simulink model "RoboBoatVU_2014_Final_Run"  (R2014a)
settings: Solver=FixedStepDiscrete  StartTime=0.0  StopTime=inf  FixedStep=.1  RelTol=1e-3
undefined symbols (not defined in the file): Com1, Com2, Com3, Com4, DiscIntNeverNeededParam, RGB24, standard
libraries: visiontextngfix x66, simulink x53, xpcseriallib x15, dspmtrx3 x14, slrtlib x3, speedgoatlib_IO102 x3, visionstatistics x2, dspstat3 x2, dspindex x2, xpcvideousblib x2, xpcvideoutillib x2, speedgoatlib x1
(part 7 of 7)

== matlab function RoboBoatVU_2014_Final_Run/Main FSM/Obstacle Navigation1/Enter Gate/Gate 2 (White & White)/MATLAB Function ==
  data: Prob input; RPM output; ColorID input; Dist input; Ang input; CurrentHeading input; GPSLat input; GPSLong input; Timer input; DesiredHeading output; gateGPS output
function [RPM,DesiredHeading,gateGPS] = navigation(Prob,ColorID,Dist,Ang,CurrentHeading,GPSLat,GPSLong,Timer)

% Function performs one buoy navigation through the start speed gates. If
% no buoys are found by the LIDAR/Vision assembly then an incremented
% turning algorithm is executed to turn by 10 degrees per increment up to 
% 90 degrees either way of the inital heading

% Written by Edward Zhu


persistent LockHeading TimeLastFound Counter Turn TurnInc gateLat gateLong

if isempty(LockHeading) && isempty(TimeLastFound) && isempty(Counter) && isempty(Turn) && isempty(TurnInc)
    LockHeading = CurrentHeading;
    TimeLastFound = 0;
    Counter = 0;
    TurnInc = 30;
    Turn = TurnInc;
    gateLat = 0;
    gateLong = 0;
end
Distance = Dist/100;
BoatWidth = 0.75;
Buffer = atan(2*BoatWidth/Distance);

RedOffset = Ang + Buffer;
WhiteOffset = Ang - Buffer;

R = 6378137;

CurLat = (floor(GPSLat/100)+mod(GPSLat,100)/60)*pi/180;
CurLong = (ceil(GPSLong/100)-mod(-GPSLong,100)/60)*pi/180;

gateHeading = (mod(CurrentHeading - Ang, 360))*pi/180;

if ColorID == 1 && Prob > 0.9
    DesiredHeading = mod(CurrentHeading - RedOffset, 360);
    RPM = 2000;
    GateFound = 1;
    TimeLastFound = Timer;
    gateLat =  asin(sin(CurLat)*cos(Distance/R) + cos(CurLat)*sin(Distance/R)*cos(gateHeading))*180/pi;
    gateLong = (CurLong + atan2(sin(gateHeading)*sin(Distance/R)*cos(CurLat),cos(Distance/R)-sin(CurLat)*sin(gateLat)))*180/pi;
elseif ColorID == 2 && Prob > 0.9
    DesiredHeading = mod(CurrentHeading - WhiteOffset, 360);
    RPM = 2000;
    GateFound = 1;
    TimeLastFound = Timer;
    gateLat =  asin(sin(CurLat)*cos(Distance/R) + cos(CurLat)*sin(Distance/R)*cos(gateHeading))*180/pi;
    gateLong = (CurLong + atan2(sin(gateHeading)*sin(Distance/R)*cos(CurLat),cos(Distance/R)-sin(CurLat)*sin(gateLat)))*180/pi;
else
    DesiredHeading = CurrentHeading;
    RPM = 0;
    GateFound = 0;
end

gateGPS = [gateLat gateLong];
TimeNoBuoys = Timer - TimeLastFound;

if GateFound == 0 && TimeNoBuoys > 15
    RPM = 0;
    DesiredHeading = mod(LockHeading - Turn, 360);
    HeadingDiff = DesiredHeading - CurrentHeading;
    gateGPS = [gateLat gateLong];
    
    if HeadingDiff > 180
        HeadingDiff = HeadingDiff - 360;
    elseif HeadingDiff < -180
        HeadingDiff = HeadingDiff + 360;
    end
    
    if HeadingDiff < 3
        Counter = Counter + 1;
    else
        Counter = 0;
    end
    
    if Counter >= 15
        Turn = Turn + TurnInc;
        Counter = 0;
        if abs(Turn) > 90
            TurnInc = -TurnInc;
        end
    end
end

== matlab function RoboBoatVU_2014_Final_Run/Main FSM/Obstacle Navigation1/GPS: Center/GPS Enabler ==
  data: Finished input; GPSMode output; OrientEnable output; ApproachEnable output
function [GPSMode, OrientEnable, ApproachEnable] =...
    GPSEnable(Finished)

%Written by Anderson Lebbad on July 22, 2013
%Last Edited: July 27, 2013
%   Removed Termination Block

%This function enables GPS tasks. First the boat orients towards the
%target, then it approaches it.


%Parse Finished signal
OrientFinished = Finished(1);


%Initialize Enablers
OrientEnable = 0;
ApproachEnable = 0;


%Switches the enable signal based on which task is flagged as done.
if OrientFinished == 0
    OrientEnable = 1;
    GPSMode = 1;
else
    ApproachEnable = 1;
    GPSMode = 2;
end

== matlab function RoboBoatVU_2014_Final_Run/Main FSM/Obstacle Navigation1/Obstacle Navigation/Dodge/Nav Logic ==
  data: CurrentHeading input; Dist input; Ang input; ObstDist output; RPM output; DesiredHeading output; Timer input; Timeout input; DodgeIncomplete output
 function [ObstDist, RPM, DesiredHeading, DodgeIncomplete] = NavLogic(CurrentHeading,...
    Dist, Ang, Timer, Timeout)

%Written by Anderson Lebbad on August 20, 2013
%Last Edited by:

%Determines the signals for driving through the buoy channel based on the
%bounding box and centroid signals from both the red and green detection
%blocks.

persistent TimeLastFound heldHeading

ObstDist = Dist / 100;

if isempty(TimeLastFound) && isempty(heldHeading)
    TimeLastFound = 0;
    heldHeading = CurrentHeading;
end

if ObstDist > 0 && ObstDist <= 2
    %Buffer for single buoy offset is the angle to twice the boat's width off of the
    %center of the buoy
    BoatWidth = .75;
    Buffer = atan(2 * BoatWidth / ObstDist) * 180 / pi;
    
    if Ang < 0
        ObstOffset = Ang + Buffer;
    else
        ObstOffset = Ang - Buffer;
    end
    
    DesiredHeading = mod(CurrentHeading + ObstOffset, 360);
    RPM = 2800;
    
    TimeLastFound = Timer;
    heldHeading = CurrentHeading;
    
    DodgeIncomplete = 1;
    
else
    DesiredHeading = heldHeading;
    RPM = 2800;
    
    if Timer-TimeLastFound < Timeout
        DodgeIncomplete = 1;
    else
        DodgeIncomplete = 0;
    end

end

== matlab function RoboBoatVU_2014_Final_Run/Main FSM/Obstacle Navigation1/Obstacle Navigation/GPS: Bee Line/Orient/Within Range ==
  data: DesiredHeading input; Finished output; Compass input
function Finished = OrientLocked(DesiredHeading, Compass)

%Written by Anderson Lebbad on July 22, 2013
%Last Edited:

%This function checks to see if the target heading has been reached and 
%sends a finished signal when it has.

HeadingDiff = DesiredHeading - Compass;

%Sets the range for the difference angle to be -180 to +180
if HeadingDiff > 180
    HeadingDiff = HeadingDiff - 360;
elseif HeadingDiff < -180
    HeadingDiff = HeadingDiff + 360;
end

%If the Heading is within 3 degrees, the angle is close enough to send a
%finished signal
if abs(HeadingDiff) < 3
    Finished = 1;
else
    Finished = 0;
end

== matlab function RoboBoatVU_2014_Final_Run/Main FSM/Shotgun Speedgate/MATLAB Function ==
  data: Heading input; LockedHeading output
function LockedHeading = HeadingLock(Heading)

persistent lock

if isempty(lock)
    lock = Heading;
end

LockedHeading = lock;

== matlab function RoboBoatVU_2014_Final_Run/Parameters/GPS Points/GPS Selector ==
  data: course input; ssGate output; rtnIn input; ssGateA input; transWptA input; obstNavStartA input; obstNavEndA input; acouLocA input; dockA input; ssGateB input; transWptB input; obstNavStartB input; obstNavEndB input; acouLocB input; dockB input; ssGateT input; transWptT input; obstNavStartT input; obstNavEndT input; acouLocT input; dockT input; transWpt output; obstNavStart output; obstNavEnd output; acouLoc output; dock output; rtnOut output
function [ssGate,transWpt,obstNavStart,obstNavEnd,acouLoc,dock,rtnOut] = ...
    GPSselector(course,rtnIn,...
    ssGateA,transWptA,obstNavStartA,obstNavEndA,acouLocA,dockA,...
    ssGateB,transWptB,obstNavStartB,obstNavEndB,acouLocB,dockB,...
    ssGateT,transWptT,obstNavStartT,obstNavEndT,acouLocT,dockT)

%Written by: Anderson Lebbad on July 18, 2013
%Last Edited: Edward Zhu on June
%   Data type mismatch addressed
%   Character conversion redundant

%Selects GPS Points to use based on input Course

%Check value of CourseStr and pass inputs accordingly

switch course
    case uint8('A')
        ssGate = ssGateA;
        transWpt = transWptA;
        obstNavStart = obstNavStartA;
        obstNavEnd = obstNavEndA;
        acouLoc = acouLocA;
        dock = dockA;
        rtnOut = rtnIn;
        
    case uint8('B')
        ssGate = ssGateB;
        transWpt = transWptB;
        obstNavStart = obstNavStartB;
        obstNavEnd = obstNavEndB;
        acouLoc = acouLocB;
        dock = dockB;
        rtnOut = rtnIn;
        
    otherwise
        ssGate = ssGateT;
        transWpt = transWptT;
        obstNavStart = obstNavStartT;
        obstNavEnd = obstNavEndT;
        acouLoc = acouLocT;
        dock = dockT;
        rtnOut = rtnIn;
end

== matlab function RoboBoatVU_2014_Final_Run/Main FSM/Acoustic Location1/GPS: Acoustic Center1/GPS Enabler ==
  data: Finished input; GPSMode output; OrientEn output; ApproachEn output
function [GPSMode, OrientEn, ApproachEn] = GPSEnable(Finished)

%Written by Anderson Lebbad on July 22, 2013
%Last Edited: July 27, 2013
%   Removed Termination Block

%This function enables GPS tasks. First the boat orients towards the
%target, then it approaches it.


%Parse Finished signal
OrientFinished = Finished(1);


%Initialize Enablers
OrientEn = 0;
ApproachEn = 0;


%Switches the enable signal based on which task is flagged as done.
if OrientFinished == 0
    OrientEn = 1;
    GPSMode = 1;
else
    ApproachEn = 1;
    GPSMode = 2;
end

== matlab function RoboBoatVU_2014_Final_Run/Main FSM/Acoustic Location1/GPS:Waypoint/Approach/Desired Heading and Distance ==
  data: Distance output; DesiredGPS input; DesiredHeading output; GPSLat input; GPSLong input
function [Distance, DesiredHeading] = Approach(DesiredGPS, GPSLat, GPSLong)

%Written by Anderson Lebbad on July 22, 2013
%Last Edited: Edward Zhu July 5, 2014

%Edit:
% Switched from great-circle distance formula to equirectangular approx and
%used mod for desired heading
% Changed calculation to use positve lat and negative long

%Orients the boat towards a target GPS point before approaching it.
%This is done to keep the approach angle minimal, so the approach
%algorithm does not circle the target and never reach it.

%Parse input GPS and convert angles to radians
CurLat = (floor(GPSLat/100)+mod(GPSLat,100)/60)*pi/180;
CurLong = (ceil(GPSLong/100)-mod(-GPSLong,100)/60)*pi/180;
DesLat = (floor(DesiredGPS(1)/100)+mod(DesiredGPS(1),100)/60)*pi/180;
DesLong = (ceil(DesiredGPS(2)/100)-mod(-DesiredGPS(2),100)/60)*pi/180;

%Difference between lats and longs
DiffLat = DesLat - CurLat;
MidLat = cos((CurLat + DesLat)/2);
DiffLong = DesLong - CurLong;

%Radius of the earth in meters
R = 6378137;

%Calculate distance using the great-circle distance formula
%Formula documented here:
%   http://www.movable-type.co.uk/scripts/latlong.html
% a = sin(DiffLat/2)^2+sin(DiffLong/2)^2*cos(CurLat)*cos(DesLat);
% c = 2*atan2(sqrt(a), sqrt(1-a));
% Distance = R*c;

%Calculating distance using equirectangular approximation since distances
%concerned are very small
a = DiffLong*MidLat;
b = DiffLat;
Distance = R*sqrt(a^2+b^2);

%Calculate initial bearing - formula documented here: 
%   http://www.movable-type.co.uk/scripts/latlong.html
y = sin(DiffLong)*cos(DesLat);
x = cos(CurLat)*sin(DesLat)-sin(CurLat)*cos(DesLat)*cos(DiffLong);
DesiredHeading = mod(atan2(y, x)*180/pi + 360, 360);

== matlab function RoboBoatVU_2014_Final_Run/Main FSM/Start Speed Gate/Buoy Decisions/Nav Logic ==
  data: Compass input; RedBBox input; GreenBBox input; RedCentroid input; GreenCentroid input; Course input; RedDist output; GreenDist output; RPM output; DesiredHeading output; Timer input; RedGain input; GreenGain input
function [RedDist, GreenDist, RPM, DesiredHeading] = NavLogic(Compass,...
    RedBBox, GreenBBox, RedCentroid, GreenCentroid, Course, Timer,RedGain,GreenGain)

%Written by Anderson Lebbad on August 20, 2013
%Last Edited by:

%Determines the signals for driving through the buoy channel based on the
%bounding box and centroid signals from both the red and green detection
%blocks.


%Initialize Outputs
RPM = 2800;
DesiredHeading = Compass;



%% First, calculate the distance each detected polyform A-0 buoy is.

%The buoy has a fixed diameter (m), the camera has a known field of view
%(which will be converted to radians for calculations) and the size of the
%frame (in pixels) is fixed
diameter = 0.3556;
FoV = 62*pi/180;
wFrame = 640;


%The bounding box passes the width of the found buoy in pixels
wRedBox = RedBBox(3);
wGreenBox = GreenBBox(3);


%The ratio of the widths in pixels corresponds to the ratio of the withs in
%meters, and the width of the frame in meters is equal to the angle of the
%field of view (in radians) multiplied by the distance it is away from the
%buoy
RedDist = (wFrame * diameter) / (wRedBox * FoV);
GreenDist = (wFrame * diameter) / (wGreenBox * FoV);



%% Second, determine angles to buoys and offset angles for steering

%Reference angle measured from bottom center of the frame (image
%coordinates are referenced to top left corner of image, with higher x
%values being more towards the right of the image, and higher y values
%being more towards the bottom of the image)
RedX = RedCentroid(1) - 320;
RedY = 480 - RedCentroid(2);
GreenX = GreenCentroid(1) - 320;
GreenY = 480 - GreenCentroid(2);


%Return angles in degrees
RedAngle = atan(RedX / RedY) * 180 / pi;
GreenAngle = atan(GreenX / GreenY) * 180 / pi;


%Buffer for single buoy offset is the angle to twice the boat's width off of the
%center of the buoy
BoatWidth = .75;
RedBuffer = atan(RedGain * BoatWidth / RedDist) * 180 / pi;
GreenBuffer = atan(GreenGain * BoatWidth / GreenDist) * 180 / pi;


%Red offset is to the right and green is to the left to stay within gates
RedOffset = RedAngle + RedBuffer;
GreenOffset = GreenAngle - GreenBuffer;



%% Third, determine whether both buoys are located and whether or not
%navigation can treat them as a pair.

%Check to see if a valid value was passed for the centroid for both the red
%and green blobs
if RedCentroid(1) == -1
    RedLocate = 0;
else
    RedLocate = 1;
end
if GreenCentroid(1) == -1
    GreenLocate = 0;
else
    GreenLocate = 1;
end


%if both are located and red is to the left of green, steer between the
%two. Otherwise, do appropriate one buoy navigation, or mark no buoys as
%found
if RedLocate == 1 && GreenLocate == 1
    if RedAngle < GreenAngle
        DesiredHeading = mod(Compass + (RedAngle + GreenAngle) / 2, 360);
        RPM = 4000;
    elseif Course == 'A'
        DesiredHeading = mod(Compass + RedOffset, 360);
    else
        DesiredHeading = mod(Compass + GreenOffset, 360);
    end
    buoysFound = 2;
elseif RedLocate == 1
    DesiredHeading = mod(Compass + RedOffset, 360);
    buoysFound = 1;
elseif GreenLocate == 1
    DesiredHeading = mod(Compass + GreenOffset, 360);
    buoysFound = 1;
else
    buoysFound = 0;
end


%% Fourth, search algorithm if no buoys are found. The search algorithm is
%designed to first hold the last heading for two seconds (in case lighting
%and focus caused the buoys to not be detected for a few frames), then to
%turn away from the last buoy position in the opposite direction of the
%other course by the angle of the field of view, and then towards the
%direction of the other course by the angle of the field of view. If a buoy
%is not found by the time this is done, the boat orients itself back in the
%direction that a buoy was last found, and slowly backs up.

%Set a persistent variables to track the last time a buoy was detected and
%heading it was at when it saw it.
persistent TimeLastFound
if isempty(TimeLastFound)
    TimeLastFound = Timer;
end
persistent HeadingLastFound
if isempty(HeadingLastFound)
    HeadingLastFound = Compass;
end


%Set a variable for tracking the time since the last buoy was found
% TimeNoBuoys = Timer - TimeLastFound;


%Set a variable for which way to initially turn during the search algorithm
%based on the course number
% if Course == 'B'
%     Turn = -FoV * 180 / pi;
% else
%     Turn = FoV * 180 / pi;
% end

%Check to see if no buoys are found, and how long it has been to determine
%what part of the search algorithm to run
if buoysFound == 0
    DesiredHeading = HeadingLastFound;
    RPM = 4000;
    %     elseif TimeNoBuoys < 20
    %         DesiredHeading = mod(HeadingLastFound + Turn, 360);
    %     elseif TimeNoBuoys < 30
    %         DesiredHeading = mod(HeadingLastFound - Turn, 360);
    %     else
    %         DesiredHeading = HeadingLastFound;
    %         RPM = -100;
    %     end
else
    TimeLastFound = Timer;
    HeadingLastFound = Compass;
end
